simulink model "test_mdl_NI"  (R2018a)
settings: Solver=VariableStepAuto  StartTime=0.0  StopTime=10.0  RelTol=1e-3
(part 18 of 24)

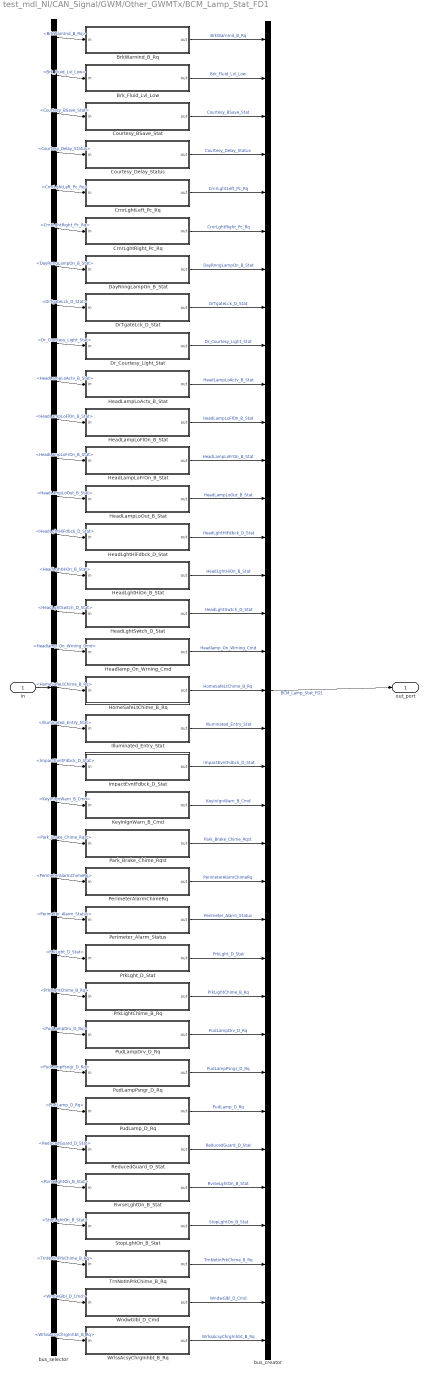
== system test_mdl_NI/CAN_Signal/GWM/Other_GWMTx/BCM_Lamp_Stat_FD1 ==
  in : Inport
  BrkWarnInd_B_Rq : Subsystem
  Brk_Fluid_Lvl_Low : Subsystem
  Courtesy_BSave_Stat : Subsystem
  Courtesy_Delay_Status : Subsystem
  CrnrLghtLeft_Pc_Rq : Subsystem
  CrnrLghtRight_Pc_Rq : Subsystem
  DayRnngLampOn_B_Stat : Subsystem
  DrTgateLck_D_Stat : Subsystem
  Dr_Courtesy_Light_Stat : Subsystem
  HeadLampLoActv_B_Stat : Subsystem
  HeadLampLoFlOn_B_Stat : Subsystem
  HeadLampLoFrOn_B_Stat : Subsystem
  HeadLampLoOut_B_Stat : Subsystem
  HeadLghtHiFdbck_D_Stat : Subsystem
  HeadLghtHiOn_B_Stat : Subsystem
  HeadLghtSwtch_D_Stat : Subsystem
  Headlamp_On_Wrning_Cmd : Subsystem
  HomeSafeLtChime_B_Rq : Subsystem
  Illuminated_Entry_Stat : Subsystem
  ImpactEvntFdbck_D_Stat : Subsystem
  KeyInIgnWarn_B_Cmd : Subsystem
  Park_Brake_Chime_Rqst : Subsystem
  PerimeterAlarmChimeRq : Subsystem
  Perimeter_Alarm_Status : Subsystem
  PrkLght_D_Stat : Subsystem
  PrkLightChime_B_Rq : Subsystem
  PudLampDrv_D_Rq : Subsystem
  PudLampPsngr_D_Rq : Subsystem
  PudLamp_D_Rq : Subsystem
  ReducedGuard_D_Stat : Subsystem
  RvrseLghtOn_B_Stat : Subsystem
  StopLghtOn_B_Stat : Subsystem
  TrnNotInPrkChime_B_Rq : Subsystem
  WndwGlbl_D_Cmd : Subsystem
  WrlssAcsyChrgInhbt_B_Rq : Subsystem
  bus_creator : BusCreator  Inputs=35
  bus_selector : BusSelector  OutputSignals=BrkWarnInd_B_Rq,Brk_Fluid_Lvl_Low,Courtesy_BSave_Stat,Courtesy_Delay_Status,CrnrLghtLeft_Pc_Rq,CrnrLghtRight_Pc_Rq,DayRnngLampOn_B_Stat,DrTgateLck_D_Stat,Dr_Courtesy_Light_Stat,HeadLampLoActv_B_Stat,HeadLampLoFlOn_B_Stat,HeadLampLoFrOn_B_Stat,HeadLampLoOut_B_Stat,HeadLghtHiFdbck_D_Stat,HeadLghtHiOn_B_Stat,HeadLghtSwtch_D_Stat,Headlamp_On_Wrning_Cmd,HomeSafeLtChime_B_Rq,Illuminated_Entry_Stat,ImpactEvntFdbck_D_Stat,KeyInIgnWarn_B_Cmd,Park_Brake_Chime_Rqst,PerimeterAlarmChimeRq,Perimeter_Alarm_Status,PrkLght_D_Stat,PrkLightChime_B_Rq,PudLampDrv_D_Rq,PudLampPsngr_D_Rq,PudLamp_D_Rq,ReducedGuard_D_Stat,RvrseLghtOn_B_Stat,StopLghtOn_B_Stat,TrnNotInPrkChime_B_Rq,WndwGlbl_D_Cmd,WrlssAcsyChrgInhbt_B_Rq
  out_port : Outport
  wires:
  bus_creator/1 -> out_port/1  "BCM_Lamp_Stat_FD1"
  BrkWarnInd_B_Rq/1(out) -> bus_creator/1  "BrkWarnInd_B_Rq"
  Brk_Fluid_Lvl_Low/1(out) -> bus_creator/2  "Brk_Fluid_Lvl_Low"
  Courtesy_BSave_Stat/1(out) -> bus_creator/3  "Courtesy_BSave_Stat"
  Courtesy_Delay_Status/1(out) -> bus_creator/4  "Courtesy_Delay_Status"
  CrnrLghtLeft_Pc_Rq/1(out) -> bus_creator/5  "CrnrLghtLeft_Pc_Rq"
  CrnrLghtRight_Pc_Rq/1(out) -> bus_creator/6  "CrnrLghtRight_Pc_Rq"
  DayRnngLampOn_B_Stat/1(out) -> bus_creator/7  "DayRnngLampOn_B_Stat"
  DrTgateLck_D_Stat/1(out) -> bus_creator/8  "DrTgateLck_D_Stat"
  Dr_Courtesy_Light_Stat/1(out) -> bus_creator/9  "Dr_Courtesy_Light_Stat"
  HeadLampLoActv_B_Stat/1(out) -> bus_creator/10  "HeadLampLoActv_B_Stat"
  HeadLampLoFlOn_B_Stat/1(out) -> bus_creator/11  "HeadLampLoFlOn_B_Stat"
  HeadLampLoFrOn_B_Stat/1(out) -> bus_creator/12  "HeadLampLoFrOn_B_Stat"
  HeadLampLoOut_B_Stat/1(out) -> bus_creator/13  "HeadLampLoOut_B_Stat"
  HeadLghtHiFdbck_D_Stat/1(out) -> bus_creator/14  "HeadLghtHiFdbck_D_Stat"
  HeadLghtHiOn_B_Stat/1(out) -> bus_creator/15  "HeadLghtHiOn_B_Stat"
  HeadLghtSwtch_D_Stat/1(out) -> bus_creator/16  "HeadLghtSwtch_D_Stat"
  Headlamp_On_Wrning_Cmd/1(out) -> bus_creator/17  "Headlamp_On_Wrning_Cmd"
  HomeSafeLtChime_B_Rq/1(out) -> bus_creator/18  "HomeSafeLtChime_B_Rq"
  Illuminated_Entry_Stat/1(out) -> bus_creator/19  "Illuminated_Entry_Stat"
  ImpactEvntFdbck_D_Stat/1(out) -> bus_creator/20  "ImpactEvntFdbck_D_Stat"
  KeyInIgnWarn_B_Cmd/1(out) -> bus_creator/21  "KeyInIgnWarn_B_Cmd"
  Park_Brake_Chime_Rqst/1(out) -> bus_creator/22  "Park_Brake_Chime_Rqst"
  PerimeterAlarmChimeRq/1(out) -> bus_creator/23  "PerimeterAlarmChimeRq"
  Perimeter_Alarm_Status/1(out) -> bus_creator/24  "Perimeter_Alarm_Status"
  PrkLght_D_Stat/1(out) -> bus_creator/25  "PrkLght_D_Stat"
  PrkLightChime_B_Rq/1(out) -> bus_creator/26  "PrkLightChime_B_Rq"
  PudLampDrv_D_Rq/1(out) -> bus_creator/27  "PudLampDrv_D_Rq"
  PudLampPsngr_D_Rq/1(out) -> bus_creator/28  "PudLampPsngr_D_Rq"
  PudLamp_D_Rq/1(out) -> bus_creator/29  "PudLamp_D_Rq"
  ReducedGuard_D_Stat/1(out) -> bus_creator/30  "ReducedGuard_D_Stat"
  RvrseLghtOn_B_Stat/1(out) -> bus_creator/31  "RvrseLghtOn_B_Stat"
  StopLghtOn_B_Stat/1(out) -> bus_creator/32  "StopLghtOn_B_Stat"
  TrnNotInPrkChime_B_Rq/1(out) -> bus_creator/33  "TrnNotInPrkChime_B_Rq"
  WndwGlbl_D_Cmd/1(out) -> bus_creator/34  "WndwGlbl_D_Cmd"
  WrlssAcsyChrgInhbt_B_Rq/1(out) -> bus_creator/35  "WrlssAcsyChrgInhbt_B_Rq"
  bus_selector/1 -> BrkWarnInd_B_Rq/1(in)  "<BrkWarnInd_B_Rq>"
  bus_selector/2 -> Brk_Fluid_Lvl_Low/1(in)  "<Brk_Fluid_Lvl_Low>"
  bus_selector/3 -> Courtesy_BSave_Stat/1(in)  "<Courtesy_BSave_Stat>"
  bus_selector/4 -> Courtesy_Delay_Status/1(in)  "<Courtesy_Delay_Status>"
  bus_selector/5 -> CrnrLghtLeft_Pc_Rq/1(in)  "<CrnrLghtLeft_Pc_Rq>"
  bus_selector/6 -> CrnrLghtRight_Pc_Rq/1(in)  "<CrnrLghtRight_Pc_Rq>"
  bus_selector/7 -> DayRnngLampOn_B_Stat/1(in)  "<DayRnngLampOn_B_Stat>"
  bus_selector/8 -> DrTgateLck_D_Stat/1(in)  "<DrTgateLck_D_Stat>"
  bus_selector/9 -> Dr_Courtesy_Light_Stat/1(in)  "<Dr_Courtesy_Light_Stat>"
  bus_selector/10 -> HeadLampLoActv_B_Stat/1(in)  "<HeadLampLoActv_B_Stat>"
  bus_selector/11 -> HeadLampLoFlOn_B_Stat/1(in)  "<HeadLampLoFlOn_B_Stat>"
  bus_selector/12 -> HeadLampLoFrOn_B_Stat/1(in)  "<HeadLampLoFrOn_B_Stat>"
  bus_selector/13 -> HeadLampLoOut_B_Stat/1(in)  "<HeadLampLoOut_B_Stat>"
  bus_selector/14 -> HeadLghtHiFdbck_D_Stat/1(in)  "<HeadLghtHiFdbck_D_Stat>"
  bus_selector/15 -> HeadLghtHiOn_B_Stat/1(in)  "<HeadLghtHiOn_B_Stat>"
  bus_selector/16 -> HeadLghtSwtch_D_Stat/1(in)  "<HeadLghtSwtch_D_Stat>"
  bus_selector/17 -> Headlamp_On_Wrning_Cmd/1(in)  "<Headlamp_On_Wrning_Cmd>"
  bus_selector/18 -> HomeSafeLtChime_B_Rq/1(in)  "<HomeSafeLtChime_B_Rq>"
  bus_selector/19 -> Illuminated_Entry_Stat/1(in)  "<Illuminated_Entry_Stat>"
  bus_selector/20 -> ImpactEvntFdbck_D_Stat/1(in)  "<ImpactEvntFdbck_D_Stat>"
  bus_selector/21 -> KeyInIgnWarn_B_Cmd/1(in)  "<KeyInIgnWarn_B_Cmd>"
  bus_selector/22 -> Park_Brake_Chime_Rqst/1(in)  "<Park_Brake_Chime_Rqst>"
  bus_selector/23 -> PerimeterAlarmChimeRq/1(in)  "<PerimeterAlarmChimeRq>"
  bus_selector/24 -> Perimeter_Alarm_Status/1(in)  "<Perimeter_Alarm_Status>"
  bus_selector/25 -> PrkLght_D_Stat/1(in)  "<PrkLght_D_Stat>"
  bus_selector/26 -> PrkLightChime_B_Rq/1(in)  "<PrkLightChime_B_Rq>"
  bus_selector/27 -> PudLampDrv_D_Rq/1(in)  "<PudLampDrv_D_Rq>"
  bus_selector/28 -> PudLampPsngr_D_Rq/1(in)  "<PudLampPsngr_D_Rq>"
  bus_selector/29 -> PudLamp_D_Rq/1(in)  "<PudLamp_D_Rq>"
  bus_selector/30 -> ReducedGuard_D_Stat/1(in)  "<ReducedGuard_D_Stat>"
  bus_selector/31 -> RvrseLghtOn_B_Stat/1(in)  "<RvrseLghtOn_B_Stat>"
  bus_selector/32 -> StopLghtOn_B_Stat/1(in)  "<StopLghtOn_B_Stat>"
  bus_selector/33 -> TrnNotInPrkChime_B_Rq/1(in)  "<TrnNotInPrkChime_B_Rq>"
  bus_selector/34 -> WndwGlbl_D_Cmd/1(in)  "<WndwGlbl_D_Cmd>"
  bus_selector/35 -> WrlssAcsyChrgInhbt_B_Rq/1(in)  "<WrlssAcsyChrgInhbt_B_Rq>"
  in/1 -> bus_selector/1

== system test_mdl_NI/CAN_Signal/GWM/Other_GWMTx/BatteryCharge_Data2_FD1 ==
  in : Inport
  ChrgCrdLck_D_Falt : Subsystem
  bus_creator : BusCreator  Inputs=1
  bus_selector : BusSelector  OutputSignals=ChrgCrdLck_D_Falt
  out_port : Outport
  wires:
  bus_creator/1 -> out_port/1  "BatteryCharge_Data2_FD1"
  ChrgCrdLck_D_Falt/1(out) -> bus_creator/1  "ChrgCrdLck_D_Falt"
  bus_selector/1 -> ChrgCrdLck_D_Falt/1(in)  "<ChrgCrdLck_D_Falt>"
  in/1 -> bus_selector/1

== system test_mdl_NI/CAN_Signal/GWM/Other_GWMTx/Battery_Mgmt_24V_FD1 ==
  in : Inport
  BattULo24Soc_Pc_Actl : Subsystem
  BattULo24State_D_Qlty : Subsystem
  BattULo24_Ah_DeltaRide : Subsystem
  BattULo24_B_Falt : Subsystem
  BattULo24_I_Actl : Subsystem
  bus_creator : BusCreator  Inputs=5
  bus_selector : BusSelector  OutputSignals=BattULo24Soc_Pc_Actl,BattULo24State_D_Qlty,BattULo24_Ah_DeltaRide,BattULo24_B_Falt,BattULo24_I_Actl
  out_port : Outport
  wires:
  bus_creator/1 -> out_port/1  "Battery_Mgmt_24V_FD1"
  BattULo24Soc_Pc_Actl/1(out) -> bus_creator/1  "BattULo24Soc_Pc_Actl"
  BattULo24State_D_Qlty/1(out) -> bus_creator/2  "BattULo24State_D_Qlty"
  BattULo24_Ah_DeltaRide/1(out) -> bus_creator/3  "BattULo24_Ah_DeltaRide"
  BattULo24_B_Falt/1(out) -> bus_creator/4  "BattULo24_B_Falt"
  BattULo24_I_Actl/1(out) -> bus_creator/5  "BattULo24_I_Actl"
  bus_selector/1 -> BattULo24Soc_Pc_Actl/1(in)  "<BattULo24Soc_Pc_Actl>"
  bus_selector/2 -> BattULo24State_D_Qlty/1(in)  "<BattULo24State_D_Qlty>"
  bus_selector/3 -> BattULo24_Ah_DeltaRide/1(in)  "<BattULo24_Ah_DeltaRide>"
  bus_selector/4 -> BattULo24_B_Falt/1(in)  "<BattULo24_B_Falt>"
  bus_selector/5 -> BattULo24_I_Actl/1(in)  "<BattULo24_I_Actl>"
  in/1 -> bus_selector/1

== system test_mdl_NI/CAN_Signal/GWM/Other_GWMTx/Battery_Mgmt_2_FD1 ==
  in : Inport
  BattULoChrg_D_Rq : Subsystem
  BattULoSrvc_T_Actl : Subsystem
  Batt_Crit_SoC_B : Subsystem
  Batt_Lo_SoC_B : Subsystem
  ChargeMode : Subsystem
  EngStrtInhbt_B_RqBatt : Subsystem
  IdleSpeedIncrease_El : Subsystem
  PeriodicElLoad_B_Stat : Subsystem
  PwSysULoFalt_D_Stat : Subsystem
  Shed_Drain_Eng_Off_B : Subsystem
  Shed_Feature_Group_ID : Subsystem
  Shed_Level_Req : Subsystem
  Shed_T_Eng_Off_B : Subsystem
  ULoRgenTestMde_B_Rq : Subsystem
  bus_creator : BusCreator  Inputs=14
  bus_selector : BusSelector  OutputSignals=BattULoChrg_D_Rq,BattULoSrvc_T_Actl,Batt_Crit_SoC_B,Batt_Lo_SoC_B,ChargeMode,EngStrtInhbt_B_RqBatt,IdleSpeedIncrease_El,PeriodicElLoad_B_Stat,PwSysULoFalt_D_Stat,Shed_Drain_Eng_Off_B,Shed_Feature_Group_ID,Shed_Level_Req,Shed_T_Eng_Off_B,ULoRgenTestMde_B_Rq
  out_port : Outport
  wires:
  bus_creator/1 -> out_port/1  "Battery_Mgmt_2_FD1"
  BattULoChrg_D_Rq/1(out) -> bus_creator/1  "BattULoChrg_D_Rq"
  BattULoSrvc_T_Actl/1(out) -> bus_creator/2  "BattULoSrvc_T_Actl"
  Batt_Crit_SoC_B/1(out) -> bus_creator/3  "Batt_Crit_SoC_B"
  Batt_Lo_SoC_B/1(out) -> bus_creator/4  "Batt_Lo_SoC_B"
  ChargeMode/1(out) -> bus_creator/5  "ChargeMode"
  EngStrtInhbt_B_RqBatt/1(out) -> bus_creator/6  "EngStrtInhbt_B_RqBatt"
  IdleSpeedIncrease_El/1(out) -> bus_creator/7  "IdleSpeedIncrease_El"
  PeriodicElLoad_B_Stat/1(out) -> bus_creator/8  "PeriodicElLoad_B_Stat"
  PwSysULoFalt_D_Stat/1(out) -> bus_creator/9  "PwSysULoFalt_D_Stat"
  Shed_Drain_Eng_Off_B/1(out) -> bus_creator/10  "Shed_Drain_Eng_Off_B"
  Shed_Feature_Group_ID/1(out) -> bus_creator/11  "Shed_Feature_Group_ID"
  Shed_Level_Req/1(out) -> bus_creator/12  "Shed_Level_Req"
  Shed_T_Eng_Off_B/1(out) -> bus_creator/13  "Shed_T_Eng_Off_B"
  ULoRgenTestMde_B_Rq/1(out) -> bus_creator/14  "ULoRgenTestMde_B_Rq"
  bus_selector/1 -> BattULoChrg_D_Rq/1(in)  "<BattULoChrg_D_Rq>"
  bus_selector/2 -> BattULoSrvc_T_Actl/1(in)  "<BattULoSrvc_T_Actl>"
  bus_selector/3 -> Batt_Crit_SoC_B/1(in)  "<Batt_Crit_SoC_B>"
  bus_selector/4 -> Batt_Lo_SoC_B/1(in)  "<Batt_Lo_SoC_B>"
  bus_selector/5 -> ChargeMode/1(in)  "<ChargeMode>"
  bus_selector/6 -> EngStrtInhbt_B_RqBatt/1(in)  "<EngStrtInhbt_B_RqBatt>"
  bus_selector/7 -> IdleSpeedIncrease_El/1(in)  "<IdleSpeedIncrease_El>"
  bus_selector/8 -> PeriodicElLoad_B_Stat/1(in)  "<PeriodicElLoad_B_Stat>"
  bus_selector/9 -> PwSysULoFalt_D_Stat/1(in)  "<PwSysULoFalt_D_Stat>"
  bus_selector/10 -> Shed_Drain_Eng_Off_B/1(in)  "<Shed_Drain_Eng_Off_B>"
  bus_selector/11 -> Shed_Feature_Group_ID/1(in)  "<Shed_Feature_Group_ID>"
  bus_selector/12 -> Shed_Level_Req/1(in)  "<Shed_Level_Req>"
  bus_selector/13 -> Shed_T_Eng_Off_B/1(in)  "<Shed_T_Eng_Off_B>"
  bus_selector/14 -> ULoRgenTestMde_B_Rq/1(in)  "<ULoRgenTestMde_B_Rq>"
  in/1 -> bus_selector/1

== system test_mdl_NI/CAN_Signal/GWM/Other_GWMTx/Battery_Mgmt_3_FD1 ==
  in : Inport
  BSBattQCapAh : Subsystem
  BSBattQDeltaRideAh : Subsystem
  BSBattSOC : Subsystem
  BSFault : Subsystem
  BattULo2_Te_Actl : Subsystem
  BattULoChrg_URate_RqMx : Subsystem
  BattULoChrg_U_RqMn : Subsystem
  BattULoChrg_U_RqMx : Subsystem
  BattULoState_D_Qlty : Subsystem
  bus_creator : BusCreator  Inputs=9
  bus_selector : BusSelector  OutputSignals=BSBattQCapAh,BSBattQDeltaRideAh,BSBattSOC,BSFault,BattULo2_Te_Actl,BattULoChrg_URate_RqMx,BattULoChrg_U_RqMn,BattULoChrg_U_RqMx,BattULoState_D_Qlty
  out_port : Outport
  wires:
  bus_creator/1 -> out_port/1  "Battery_Mgmt_3_FD1"
  BSBattQCapAh/1(out) -> bus_creator/1  "BSBattQCapAh"
  BSBattQDeltaRideAh/1(out) -> bus_creator/2  "BSBattQDeltaRideAh"
  BSBattSOC/1(out) -> bus_creator/3  "BSBattSOC"
  BSFault/1(out) -> bus_creator/4  "BSFault"
  BattULo2_Te_Actl/1(out) -> bus_creator/5  "BattULo2_Te_Actl"
  BattULoChrg_URate_RqMx/1(out) -> bus_creator/6  "BattULoChrg_URate_RqMx"
  BattULoChrg_U_RqMn/1(out) -> bus_creator/7  "BattULoChrg_U_RqMn"
  BattULoChrg_U_RqMx/1(out) -> bus_creator/8  "BattULoChrg_U_RqMx"
  BattULoState_D_Qlty/1(out) -> bus_creator/9  "BattULoState_D_Qlty"
  bus_selector/1 -> BSBattQCapAh/1(in)  "<BSBattQCapAh>"
  bus_selector/2 -> BSBattQDeltaRideAh/1(in)  "<BSBattQDeltaRideAh>"
  bus_selector/3 -> BSBattSOC/1(in)  "<BSBattSOC>"
  bus_selector/4 -> BSFault/1(in)  "<BSFault>"
  bus_selector/5 -> BattULo2_Te_Actl/1(in)  "<BattULo2_Te_Actl>"
  bus_selector/6 -> BattULoChrg_URate_RqMx/1(in)  "<BattULoChrg_URate_RqMx>"
  bus_selector/7 -> BattULoChrg_U_RqMn/1(in)  "<BattULoChrg_U_RqMn>"
  bus_selector/8 -> BattULoChrg_U_RqMx/1(in)  "<BattULoChrg_U_RqMx>"
  bus_selector/9 -> BattULoState_D_Qlty/1(in)  "<BattULoState_D_Qlty>"
  in/1 -> bus_selector/1

== system test_mdl_NI/CAN_Signal/GWM/Other_GWMTx/Battery_Mgmt_4_FD1 ==
  in : Inport
  BattULoAuxSoc_Pc_Actl : Subsystem
  BattULoAux_B_Falt : Subsystem
  BattULoAux_D_Qlty : Subsystem
  BattULoAux_I_Actl : Subsystem
  BattULoAux_U_Actl : Subsystem
  BattULoCrnkBelt_U_Pred : Subsystem
  BattULoCrnkStrt_U_Pred : Subsystem
  bus_creator : BusCreator  Inputs=7
  bus_selector : BusSelector  OutputSignals=BattULoAuxSoc_Pc_Actl,BattULoAux_B_Falt,BattULoAux_D_Qlty,BattULoAux_I_Actl,BattULoAux_U_Actl,BattULoCrnkBelt_U_Pred,BattULoCrnkStrt_U_Pred
  out_port : Outport
  wires:
  bus_creator/1 -> out_port/1  "Battery_Mgmt_4_FD1"
  BattULoAuxSoc_Pc_Actl/1(out) -> bus_creator/1  "BattULoAuxSoc_Pc_Actl"
  BattULoAux_B_Falt/1(out) -> bus_creator/2  "BattULoAux_B_Falt"
  BattULoAux_D_Qlty/1(out) -> bus_creator/3  "BattULoAux_D_Qlty"
  BattULoAux_I_Actl/1(out) -> bus_creator/4  "BattULoAux_I_Actl"
  BattULoAux_U_Actl/1(out) -> bus_creator/5  "BattULoAux_U_Actl"
  BattULoCrnkBelt_U_Pred/1(out) -> bus_creator/6  "BattULoCrnkBelt_U_Pred"
  BattULoCrnkStrt_U_Pred/1(out) -> bus_creator/7  "BattULoCrnkStrt_U_Pred"
  bus_selector/1 -> BattULoAuxSoc_Pc_Actl/1(in)  "<BattULoAuxSoc_Pc_Actl>"
  bus_selector/2 -> BattULoAux_B_Falt/1(in)  "<BattULoAux_B_Falt>"
  bus_selector/3 -> BattULoAux_D_Qlty/1(in)  "<BattULoAux_D_Qlty>"
  bus_selector/4 -> BattULoAux_I_Actl/1(in)  "<BattULoAux_I_Actl>"
  bus_selector/5 -> BattULoAux_U_Actl/1(in)  "<BattULoAux_U_Actl>"
  bus_selector/6 -> BattULoCrnkBelt_U_Pred/1(in)  "<BattULoCrnkBelt_U_Pred>"
  bus_selector/7 -> BattULoCrnkStrt_U_Pred/1(in)  "<BattULoCrnkStrt_U_Pred>"
  in/1 -> bus_selector/1

== system test_mdl_NI/CAN_Signal/GWM/Other_GWMTx/Battery_Traction_1_FD1 ==
  in : Inport
  BattTracMil_D_Rq : Subsystem
  BattTracOffFst_D_Actl : Subsystem
  BattTracOff_B_Actl : Subsystem
  BattTrac_I_Actl : Subsystem
  BattTrac_U_Actl : Subsystem
  BattTrac_U_LimHi : Subsystem
  BattTrac_U_LimLo : Subsystem
  VehStrtInhbt_B_RqBatt : Subsystem
  bus_creator : BusCreator  Inputs=8
  bus_selector : BusSelector  OutputSignals=BattTracMil_D_Rq,BattTracOffFst_D_Actl,BattTracOff_B_Actl,BattTrac_I_Actl,BattTrac_U_Actl,BattTrac_U_LimHi,BattTrac_U_LimLo,VehStrtInhbt_B_RqBatt
  out_port : Outport
  wires:
  bus_creator/1 -> out_port/1  "Battery_Traction_1_FD1"
  BattTracMil_D_Rq/1(out) -> bus_creator/1  "BattTracMil_D_Rq"
  BattTracOffFst_D_Actl/1(out) -> bus_creator/2  "BattTracOffFst_D_Actl"
  BattTracOff_B_Actl/1(out) -> bus_creator/3  "BattTracOff_B_Actl"
  BattTrac_I_Actl/1(out) -> bus_creator/4  "BattTrac_I_Actl"
  BattTrac_U_Actl/1(out) -> bus_creator/5  "BattTrac_U_Actl"
  BattTrac_U_LimHi/1(out) -> bus_creator/6  "BattTrac_U_LimHi"
  BattTrac_U_LimLo/1(out) -> bus_creator/7  "BattTrac_U_LimLo"
  VehStrtInhbt_B_RqBatt/1(out) -> bus_creator/8  "VehStrtInhbt_B_RqBatt"
  bus_selector/1 -> BattTracMil_D_Rq/1(in)  "<BattTracMil_D_Rq>"
  bus_selector/2 -> BattTracOffFst_D_Actl/1(in)  "<BattTracOffFst_D_Actl>"
  bus_selector/3 -> BattTracOff_B_Actl/1(in)  "<BattTracOff_B_Actl>"
  bus_selector/4 -> BattTrac_I_Actl/1(in)  "<BattTrac_I_Actl>"
  bus_selector/5 -> BattTrac_U_Actl/1(in)  "<BattTrac_U_Actl>"
  bus_selector/6 -> BattTrac_U_LimHi/1(in)  "<BattTrac_U_LimHi>"
  bus_selector/7 -> BattTrac_U_LimLo/1(in)  "<BattTrac_U_LimLo>"
  bus_selector/8 -> VehStrtInhbt_B_RqBatt/1(in)  "<VehStrtInhbt_B_RqBatt>"
  in/1 -> bus_selector/1

== system test_mdl_NI/CAN_Signal/GWM/Other_GWMTx/Battery_Traction_3_FD1 ==
  in : Inport
  BattTracClnt_Te_Actl : Subsystem
  BattTracSoc_Pc_LimHi : Subsystem
  BattTracSoc_Pc_LimLo : Subsystem
  BattTracSoc_Pc_MnPrtct : Subsystem
  BattTracSoc_Pc_MxPrtct : Subsystem
  BattTracSrvcRqd_B_Rq : Subsystem
  BattTracWarnLamp_B_Rq : Subsystem
  bus_creator : BusCreator  Inputs=7
  bus_selector : BusSelector  OutputSignals=BattTracClnt_Te_Actl,BattTracSoc_Pc_LimHi,BattTracSoc_Pc_LimLo,BattTracSoc_Pc_MnPrtct,BattTracSoc_Pc_MxPrtct,BattTracSrvcRqd_B_Rq,BattTracWarnLamp_B_Rq
  out_port : Outport
  wires:
  bus_creator/1 -> out_port/1  "Battery_Traction_3_FD1"
  BattTracClnt_Te_Actl/1(out) -> bus_creator/1  "BattTracClnt_Te_Actl"
  BattTracSoc_Pc_LimHi/1(out) -> bus_creator/2  "BattTracSoc_Pc_LimHi"
  BattTracSoc_Pc_LimLo/1(out) -> bus_creator/3  "BattTracSoc_Pc_LimLo"
  BattTracSoc_Pc_MnPrtct/1(out) -> bus_creator/4  "BattTracSoc_Pc_MnPrtct"
  BattTracSoc_Pc_MxPrtct/1(out) -> bus_creator/5  "BattTracSoc_Pc_MxPrtct"
  BattTracSrvcRqd_B_Rq/1(out) -> bus_creator/6  "BattTracSrvcRqd_B_Rq"
  BattTracWarnLamp_B_Rq/1(out) -> bus_creator/7  "BattTracWarnLamp_B_Rq"
  bus_selector/1 -> BattTracClnt_Te_Actl/1(in)  "<BattTracClnt_Te_Actl>"
  bus_selector/2 -> BattTracSoc_Pc_LimHi/1(in)  "<BattTracSoc_Pc_LimHi>"
  bus_selector/3 -> BattTracSoc_Pc_LimLo/1(in)  "<BattTracSoc_Pc_LimLo>"
  bus_selector/4 -> BattTracSoc_Pc_MnPrtct/1(in)  "<BattTracSoc_Pc_MnPrtct>"
  bus_selector/5 -> BattTracSoc_Pc_MxPrtct/1(in)  "<BattTracSoc_Pc_MxPrtct>"
  bus_selector/6 -> BattTracSrvcRqd_B_Rq/1(in)  "<BattTracSrvcRqd_B_Rq>"
  bus_selector/7 -> BattTracWarnLamp_B_Rq/1(in)  "<BattTracWarnLamp_B_Rq>"
  in/1 -> bus_selector/1

== system test_mdl_NI/CAN_Signal/GWM/Other_GWMTx/Battery_Traction_4_FD1 ==
  in : Inport
  BattTracDiagClr_B_Rq : Subsystem
  BattTracSoc2_Pc_Actl : Subsystem
  BattTrac_Te_Actl : Subsystem
  bus_creator : BusCreator  Inputs=3
  bus_selector : BusSelector  OutputSignals=BattTracDiagClr_B_Rq,BattTracSoc2_Pc_Actl,BattTrac_Te_Actl
  out_port : Outport
  wires:
  bus_creator/1 -> out_port/1  "Battery_Traction_4_FD1"
  BattTracDiagClr_B_Rq/1(out) -> bus_creator/1  "BattTracDiagClr_B_Rq"
  BattTracSoc2_Pc_Actl/1(out) -> bus_creator/2  "BattTracSoc2_Pc_Actl"
  BattTrac_Te_Actl/1(out) -> bus_creator/3  "BattTrac_Te_Actl"
  bus_selector/1 -> BattTracDiagClr_B_Rq/1(in)  "<BattTracDiagClr_B_Rq>"
  bus_selector/2 -> BattTracSoc2_Pc_Actl/1(in)  "<BattTracSoc2_Pc_Actl>"
  bus_selector/3 -> BattTrac_Te_Actl/1(in)  "<BattTrac_Te_Actl>"
  in/1 -> bus_selector/1

== system test_mdl_NI/CAN_Signal/GWM/Other_GWMTx/Battery_Traction_5_FD1 ==
  in : Inport
  BattTrac2_Pw_ChrgInst : Subsystem
  BattTrac2_Pw_DchrgInst : Subsystem
  BattTrac2_Pw_LimChrg : Subsystem
  BattTrac2_Pw_LimDchrg : Subsystem
  bus_creator : BusCreator  Inputs=4
  bus_selector : BusSelector  OutputSignals=BattTrac2_Pw_ChrgInst,BattTrac2_Pw_DchrgInst,BattTrac2_Pw_LimChrg,BattTrac2_Pw_LimDchrg
  out_port : Outport
  wires:
  bus_creator/1 -> out_port/1  "Battery_Traction_5_FD1"
  BattTrac2_Pw_ChrgInst/1(out) -> bus_creator/1  "BattTrac2_Pw_ChrgInst"
  BattTrac2_Pw_DchrgInst/1(out) -> bus_creator/2  "BattTrac2_Pw_DchrgInst"
  BattTrac2_Pw_LimChrg/1(out) -> bus_creator/3  "BattTrac2_Pw_LimChrg"
  BattTrac2_Pw_LimDchrg/1(out) -> bus_creator/4  "BattTrac2_Pw_LimDchrg"
  bus_selector/1 -> BattTrac2_Pw_ChrgInst/1(in)  "<BattTrac2_Pw_ChrgInst>"
  bus_selector/2 -> BattTrac2_Pw_DchrgInst/1(in)  "<BattTrac2_Pw_DchrgInst>"
  bus_selector/3 -> BattTrac2_Pw_LimChrg/1(in)  "<BattTrac2_Pw_LimChrg>"
  bus_selector/4 -> BattTrac2_Pw_LimDchrg/1(in)  "<BattTrac2_Pw_LimDchrg>"
  in/1 -> bus_selector/1

== system test_mdl_NI/CAN_Signal/GWM/Other_GWMTx/Battery_Traction_6_FD1 ==
  in : Inport
  BattTracClntPmp_D_Stat : Subsystem
  BattTracCnnct_D_Cmd : Subsystem
  BattTracDcdcDis_B_Rq : Subsystem
  BattTracDelta_Te_Actl : Subsystem
  BattTracHvilOpen_B_Stat : Subsystem
  HtrnClntPump_D_Stat : Subsystem
  bus_creator : BusCreator  Inputs=6
  bus_selector : BusSelector  OutputSignals=BattTracClntPmp_D_Stat,BattTracCnnct_D_Cmd,BattTracDcdcDis_B_Rq,BattTracDelta_Te_Actl,BattTracHvilOpen_B_Stat,HtrnClntPump_D_Stat
  out_port : Outport
  wires:
  bus_creator/1 -> out_port/1  "Battery_Traction_6_FD1"
  BattTracClntPmp_D_Stat/1(out) -> bus_creator/1  "BattTracClntPmp_D_Stat"
  BattTracCnnct_D_Cmd/1(out) -> bus_creator/2  "BattTracCnnct_D_Cmd"
  BattTracDcdcDis_B_Rq/1(out) -> bus_creator/3  "BattTracDcdcDis_B_Rq"
  BattTracDelta_Te_Actl/1(out) -> bus_creator/4  "BattTracDelta_Te_Actl"
  BattTracHvilOpen_B_Stat/1(out) -> bus_creator/5  "BattTracHvilOpen_B_Stat"
  HtrnClntPump_D_Stat/1(out) -> bus_creator/6  "HtrnClntPump_D_Stat"
  bus_selector/1 -> BattTracClntPmp_D_Stat/1(in)  "<BattTracClntPmp_D_Stat>"
  bus_selector/2 -> BattTracCnnct_D_Cmd/1(in)  "<BattTracCnnct_D_Cmd>"
  bus_selector/3 -> BattTracDcdcDis_B_Rq/1(in)  "<BattTracDcdcDis_B_Rq>"
  bus_selector/4 -> BattTracDelta_Te_Actl/1(in)  "<BattTracDelta_Te_Actl>"
  bus_selector/5 -> BattTracHvilOpen_B_Stat/1(in)  "<BattTracHvilOpen_B_Stat>"
  bus_selector/6 -> HtrnClntPump_D_Stat/1(in)  "<HtrnClntPump_D_Stat>"
  in/1 -> bus_selector/1

== system test_mdl_NI/CAN_Signal/GWM/Other_GWMTx/BodyInfo_3_FD1 ==
  in : Inport
  Backlit_LED_Status : Subsystem
  BodySrvcRqd_B_Rq : Subsystem
  CrashEvnt_D_Stat : Subsystem
  Day_Night_Status : Subsystem
  Delay_Accy : Subsystem
  DimmingLvlEvnt_No_Actl : Subsystem
  Dimming_Lvl : Subsystem
  DrStatDrvErrCnt_B_Stat : Subsystem
  DrStatDrv_B_Actl : Subsystem
  DrStatHood_B_Actl : Subsystem
  DrStatInnrTgate_B_Actl : Subsystem
  DrStatPsngr_B_Actl : Subsystem
  DrStatRl_B_Actl : Subsystem
  DrStatRr_B_Actl : Subsystem
  DrStatTgate_B_Actl : Subsystem
  FogLghtFrontOn_B_Stat : Subsystem
  FogLghtRearOn_B_Stat : Subsystem
  FuelPmpInhbt_B_Stat : Subsystem
  IgnKeyType_D_Actl : Subsystem
  Ignition_Status : Subsystem
  Key_In_Ignition_Stat : Subsystem
  LifeCycMde_D_Actl : Subsystem
  Litval : Subsystem
  Parklamp_Status : Subsystem
  PrkBrkActv_B_Actl : Subsystem
  Remote_Start_Status : Subsystem
  TurnLghtLeftOn_B_Stat : Subsystem
  TurnLghtLeft_D_Rq : Subsystem
  TurnLghtRightOn_B_Stat : Subsystem
  TurnLghtRight_D_Rq : Subsystem
  ValetMode_D_Mem : Subsystem
  bus_creator : BusCreator  Inputs=31
  bus_selector : BusSelector  OutputSignals=Backlit_LED_Status,BodySrvcRqd_B_Rq,CrashEvnt_D_Stat,Day_Night_Status,Delay_Accy,DimmingLvlEvnt_No_Actl,Dimming_Lvl,DrStatDrvErrCnt_B_Stat,DrStatDrv_B_Actl,DrStatHood_B_Actl,DrStatInnrTgate_B_Actl,DrStatPsngr_B_Actl,DrStatRl_B_Actl,DrStatRr_B_Actl,DrStatTgate_B_Actl,FogLghtFrontOn_B_Stat,FogLghtRearOn_B_Stat,FuelPmpInhbt_B_Stat,IgnKeyType_D_Actl,Ignition_Status,Key_In_Ignition_Stat,LifeCycMde_D_Actl,Litval,Parklamp_Status,PrkBrkActv_B_Actl,Remote_Start_Status,TurnLghtLeftOn_B_Stat,TurnLghtLeft_D_Rq,TurnLghtRightOn_B_Stat,TurnLghtRight_D_Rq,ValetMode_D_Mem
  out_port : Outport
  wires:
  bus_creator/1 -> out_port/1  "BodyInfo_3_FD1"
  Backlit_LED_Status/1(out) -> bus_creator/1  "Backlit_LED_Status"
  BodySrvcRqd_B_Rq/1(out) -> bus_creator/2  "BodySrvcRqd_B_Rq"
  CrashEvnt_D_Stat/1(out) -> bus_creator/3  "CrashEvnt_D_Stat"
  Day_Night_Status/1(out) -> bus_creator/4  "Day_Night_Status"
  Delay_Accy/1(out) -> bus_creator/5  "Delay_Accy"
  DimmingLvlEvnt_No_Actl/1(out) -> bus_creator/6  "DimmingLvlEvnt_No_Actl"
  Dimming_Lvl/1(out) -> bus_creator/7  "Dimming_Lvl"
  DrStatDrvErrCnt_B_Stat/1(out) -> bus_creator/8  "DrStatDrvErrCnt_B_Stat"
  DrStatDrv_B_Actl/1(out) -> bus_creator/9  "DrStatDrv_B_Actl"
  DrStatHood_B_Actl/1(out) -> bus_creator/10  "DrStatHood_B_Actl"
  DrStatInnrTgate_B_Actl/1(out) -> bus_creator/11  "DrStatInnrTgate_B_Actl"
  DrStatPsngr_B_Actl/1(out) -> bus_creator/12  "DrStatPsngr_B_Actl"
  DrStatRl_B_Actl/1(out) -> bus_creator/13  "DrStatRl_B_Actl"
  DrStatRr_B_Actl/1(out) -> bus_creator/14  "DrStatRr_B_Actl"
  DrStatTgate_B_Actl/1(out) -> bus_creator/15  "DrStatTgate_B_Actl"
  FogLghtFrontOn_B_Stat/1(out) -> bus_creator/16  "FogLghtFrontOn_B_Stat"
  FogLghtRearOn_B_Stat/1(out) -> bus_creator/17  "FogLghtRearOn_B_Stat"
  FuelPmpInhbt_B_Stat/1(out) -> bus_creator/18  "FuelPmpInhbt_B_Stat"
  IgnKeyType_D_Actl/1(out) -> bus_creator/19  "IgnKeyType_D_Actl"
  Ignition_Status/1(out) -> bus_creator/20  "Ignition_Status"
  Key_In_Ignition_Stat/1(out) -> bus_creator/21  "Key_In_Ignition_Stat"
  LifeCycMde_D_Actl/1(out) -> bus_creator/22  "LifeCycMde_D_Actl"
  Litval/1(out) -> bus_creator/23  "Litval"
  Parklamp_Status/1(out) -> bus_creator/24  "Parklamp_Status"
  PrkBrkActv_B_Actl/1(out) -> bus_creator/25  "PrkBrkActv_B_Actl"
  Remote_Start_Status/1(out) -> bus_creator/26  "Remote_Start_Status"
  TurnLghtLeftOn_B_Stat/1(out) -> bus_creator/27  "TurnLghtLeftOn_B_Stat"
  TurnLghtLeft_D_Rq/1(out) -> bus_creator/28  "TurnLghtLeft_D_Rq"
  TurnLghtRightOn_B_Stat/1(out) -> bus_creator/29  "TurnLghtRightOn_B_Stat"
  TurnLghtRight_D_Rq/1(out) -> bus_creator/30  "TurnLghtRight_D_Rq"
  ValetMode_D_Mem/1(out) -> bus_creator/31  "ValetMode_D_Mem"
  bus_selector/1 -> Backlit_LED_Status/1(in)  "<Backlit_LED_Status>"
  bus_selector/2 -> BodySrvcRqd_B_Rq/1(in)  "<BodySrvcRqd_B_Rq>"
  bus_selector/3 -> CrashEvnt_D_Stat/1(in)  "<CrashEvnt_D_Stat>"
  bus_selector/4 -> Day_Night_Status/1(in)  "<Day_Night_Status>"
  bus_selector/5 -> Delay_Accy/1(in)  "<Delay_Accy>"
  bus_selector/6 -> DimmingLvlEvnt_No_Actl/1(in)  "<DimmingLvlEvnt_No_Actl>"
  bus_selector/7 -> Dimming_Lvl/1(in)  "<Dimming_Lvl>"
  bus_selector/8 -> DrStatDrvErrCnt_B_Stat/1(in)  "<DrStatDrvErrCnt_B_Stat>"
  bus_selector/9 -> DrStatDrv_B_Actl/1(in)  "<DrStatDrv_B_Actl>"
  bus_selector/10 -> DrStatHood_B_Actl/1(in)  "<DrStatHood_B_Actl>"
  bus_selector/11 -> DrStatInnrTgate_B_Actl/1(in)  "<DrStatInnrTgate_B_Actl>"
  bus_selector/12 -> DrStatPsngr_B_Actl/1(in)  "<DrStatPsngr_B_Actl>"
  bus_selector/13 -> DrStatRl_B_Actl/1(in)  "<DrStatRl_B_Actl>"
  bus_selector/14 -> DrStatRr_B_Actl/1(in)  "<DrStatRr_B_Actl>"
  bus_selector/15 -> DrStatTgate_B_Actl/1(in)  "<DrStatTgate_B_Actl>"
  bus_selector/16 -> FogLghtFrontOn_B_Stat/1(in)  "<FogLghtFrontOn_B_Stat>"
  bus_selector/17 -> FogLghtRearOn_B_Stat/1(in)  "<FogLghtRearOn_B_Stat>"
  bus_selector/18 -> FuelPmpInhbt_B_Stat/1(in)  "<FuelPmpInhbt_B_Stat>"
  bus_selector/19 -> IgnKeyType_D_Actl/1(in)  "<IgnKeyType_D_Actl>"
  bus_selector/20 -> Ignition_Status/1(in)  "<Ignition_Status>"
  bus_selector/21 -> Key_In_Ignition_Stat/1(in)  "<Key_In_Ignition_Stat>"
  bus_selector/22 -> LifeCycMde_D_Actl/1(in)  "<LifeCycMde_D_Actl>"
  bus_selector/23 -> Litval/1(in)  "<Litval>"
  bus_selector/24 -> Parklamp_Status/1(in)  "<Parklamp_Status>"
  bus_selector/25 -> PrkBrkActv_B_Actl/1(in)  "<PrkBrkActv_B_Actl>"
  bus_selector/26 -> Remote_Start_Status/1(in)  "<Remote_Start_Status>"
  bus_selector/27 -> TurnLghtLeftOn_B_Stat/1(in)  "<TurnLghtLeftOn_B_Stat>"
  bus_selector/28 -> TurnLghtLeft_D_Rq/1(in)  "<TurnLghtLeft_D_Rq>"
  bus_selector/29 -> TurnLghtRightOn_B_Stat/1(in)  "<TurnLghtRightOn_B_Stat>"
  bus_selector/30 -> TurnLghtRight_D_Rq/1(in)  "<TurnLghtRight_D_Rq>"
  bus_selector/31 -> ValetMode_D_Mem/1(in)  "<ValetMode_D_Mem>"
  in/1 -> bus_selector/1

== system test_mdl_NI/CAN_Signal/GWM/Other_GWMTx/Body_Info_10_FD1 ==
  in : Inport
  GenericSwtch1_No_Actl : Subsystem
  GenericSwtch2_No_Actl : Subsystem
  GenericSwtch3_No_Actl : Subsystem
  bus_creator : BusCreator  Inputs=3
  bus_selector : BusSelector  OutputSignals=GenericSwtch1_No_Actl,GenericSwtch2_No_Actl,GenericSwtch3_No_Actl
  out_port : Outport
  wires:
  bus_creator/1 -> out_port/1  "Body_Info_10_FD1"
  GenericSwtch1_No_Actl/1(out) -> bus_creator/1  "GenericSwtch1_No_Actl"
  GenericSwtch2_No_Actl/1(out) -> bus_creator/2  "GenericSwtch2_No_Actl"
  GenericSwtch3_No_Actl/1(out) -> bus_creator/3  "GenericSwtch3_No_Actl"
  bus_selector/1 -> GenericSwtch1_No_Actl/1(in)  "<GenericSwtch1_No_Actl>"
  bus_selector/2 -> GenericSwtch2_No_Actl/1(in)  "<GenericSwtch2_No_Actl>"
  bus_selector/3 -> GenericSwtch3_No_Actl/1(in)  "<GenericSwtch3_No_Actl>"
  in/1 -> bus_selector/1

== system test_mdl_NI/CAN_Signal/GWM/Other_GWMTx/Body_Info_4_FD1 ==
  in : Inport
  BattULo_I_Actl : Subsystem
  BattULo_U_Actl : Subsystem
  BrkTrnShifLck_B_Stat : Subsystem
  DcacElPw_D_Rq : Subsystem
  DriverCrankingReq : Subsystem
  EngOff_T_Actl : Subsystem
  FuelPumpPwr_D_Stat : Subsystem
  PrkLckCtlAvail_T_Stat : Subsystem
  PrkLckCtlMsgTxt_D_Rq : Subsystem
  PrkLckCtlTow_B_Enbl : Subsystem
  PrkLckCtlUnlck_D_Stat : Subsystem
  PrkLckCtl_B_Enbl : Subsystem
  PtLatchActv_B_RqBcm : Subsystem
  ReFuelSwtchStat_D_Actl : Subsystem
  bus_creator : BusCreator  Inputs=15
  bus_selector : BusSelector  OutputSignals=BattULo_I_Actl,BattULo_U_Actl,BrkTrnShifLck_B_Stat,DcacElPw_D_Rq,DriverCrankingReq,EngOff_T_Actl,FuelPumpPwr_D_Stat,PrkLckCtlAvail_T_Stat,PrkLckCtlMsgTxt_D_Rq,PrkLckCtlTow_B_Enbl,PrkLckCtlUnlck_D_Stat,PrkLckCtl_B_Enbl,PtLatchActv_B_RqBcm,ReFuelSwtchStat_D_Actl,immoSecureIdleMode
  immoSecureIdleMode : Subsystem
  out_port : Outport
  wires:
  bus_creator/1 -> out_port/1  "Body_Info_4_FD1"
  BattULo_I_Actl/1(out) -> bus_creator/1  "BattULo_I_Actl"
  BattULo_U_Actl/1(out) -> bus_creator/2  "BattULo_U_Actl"
  BrkTrnShifLck_B_Stat/1(out) -> bus_creator/3  "BrkTrnShifLck_B_Stat"
  DcacElPw_D_Rq/1(out) -> bus_creator/4  "DcacElPw_D_Rq"
  DriverCrankingReq/1(out) -> bus_creator/5  "DriverCrankingReq"
  EngOff_T_Actl/1(out) -> bus_creator/6  "EngOff_T_Actl"
  FuelPumpPwr_D_Stat/1(out) -> bus_creator/7  "FuelPumpPwr_D_Stat"
  PrkLckCtlAvail_T_Stat/1(out) -> bus_creator/8  "PrkLckCtlAvail_T_Stat"
  PrkLckCtlMsgTxt_D_Rq/1(out) -> bus_creator/9  "PrkLckCtlMsgTxt_D_Rq"
  PrkLckCtlTow_B_Enbl/1(out) -> bus_creator/10  "PrkLckCtlTow_B_Enbl"
  PrkLckCtlUnlck_D_Stat/1(out) -> bus_creator/11  "PrkLckCtlUnlck_D_Stat"
  PrkLckCtl_B_Enbl/1(out) -> bus_creator/12  "PrkLckCtl_B_Enbl"
  PtLatchActv_B_RqBcm/1(out) -> bus_creator/13  "PtLatchActv_B_RqBcm"
  ReFuelSwtchStat_D_Actl/1(out) -> bus_creator/14  "ReFuelSwtchStat_D_Actl"
  immoSecureIdleMode/1(out) -> bus_creator/15  "immoSecureIdleMode"
  bus_selector/1 -> BattULo_I_Actl/1(in)  "<BattULo_I_Actl>"
  bus_selector/2 -> BattULo_U_Actl/1(in)  "<BattULo_U_Actl>"
  bus_selector/3 -> BrkTrnShifLck_B_Stat/1(in)  "<BrkTrnShifLck_B_Stat>"
  bus_selector/4 -> DcacElPw_D_Rq/1(in)  "<DcacElPw_D_Rq>"
  bus_selector/5 -> DriverCrankingReq/1(in)  "<DriverCrankingReq>"
  bus_selector/6 -> EngOff_T_Actl/1(in)  "<EngOff_T_Actl>"
  bus_selector/7 -> FuelPumpPwr_D_Stat/1(in)  "<FuelPumpPwr_D_Stat>"
  bus_selector/8 -> PrkLckCtlAvail_T_Stat/1(in)  "<PrkLckCtlAvail_T_Stat>"
  bus_selector/9 -> PrkLckCtlMsgTxt_D_Rq/1(in)  "<PrkLckCtlMsgTxt_D_Rq>"
  bus_selector/10 -> PrkLckCtlTow_B_Enbl/1(in)  "<PrkLckCtlTow_B_Enbl>"
  bus_selector/11 -> PrkLckCtlUnlck_D_Stat/1(in)  "<PrkLckCtlUnlck_D_Stat>"
  bus_selector/12 -> PrkLckCtl_B_Enbl/1(in)  "<PrkLckCtl_B_Enbl>"
  bus_selector/13 -> PtLatchActv_B_RqBcm/1(in)  "<PtLatchActv_B_RqBcm>"
  bus_selector/14 -> ReFuelSwtchStat_D_Actl/1(in)  "<ReFuelSwtchStat_D_Actl>"
  bus_selector/15 -> immoSecureIdleMode/1(in)  "<immoSecureIdleMode>"
  in/1 -> bus_selector/1

== system test_mdl_NI/CAN_Signal/GWM/Other_GWMTx/Body_Info_6_FD1 ==
  in : Inport
  DrLatchMsgTxt_D_Rq : Subsystem
  ElPwPoint_D_Rq : Subsystem
  HeadLghtHiPrmsn_D_Stat : Subsystem
  IgnPsswrdDsply_B_Rq : Subsystem
  KeyAdmnTot_No_Cnt : Subsystem
  KeyMykeyTot_No_Cnt : Subsystem
  Keycode_Status : Subsystem
  PEBackupSlot_Stats : Subsystem
  PoliceIdlMde_D_Stat : Subsystem
  PrmtrAlrmEvnt_D_Stat : Subsystem
  PrsnlDevcChrgEnbl_B_Rq : Subsystem
  SecurityMsgTxt_D_Rq : Subsystem
  SteWhlLckMsgTxt_D_Rq : Subsystem
  TracKeyMde_D_Stat : Subsystem
  bus_creator : BusCreator  Inputs=15
  bus_selector : BusSelector  OutputSignals=DrLatchMsgTxt_D_Rq,ElPwPoint_D_Rq,HeadLghtHiPrmsn_D_Stat,IgnPsswrdDsply_B_Rq,KeyAdmnTot_No_Cnt,KeyMykeyTot_No_Cnt,Keycode_Status,PEBackupSlot_Stats,PoliceIdlMde_D_Stat,PrmtrAlrmEvnt_D_Stat,PrsnlDevcChrgEnbl_B_Rq,SecurityMsgTxt_D_Rq,SteWhlLckMsgTxt_D_Rq,TracKeyMde_D_Stat,immoMsgTxt_D_Rq
  immoMsgTxt_D_Rq : Subsystem
  out_port : Outport
  wires:
  bus_creator/1 -> out_port/1  "Body_Info_6_FD1"
  DrLatchMsgTxt_D_Rq/1(out) -> bus_creator/1  "DrLatchMsgTxt_D_Rq"
  ElPwPoint_D_Rq/1(out) -> bus_creator/2  "ElPwPoint_D_Rq"
  HeadLghtHiPrmsn_D_Stat/1(out) -> bus_creator/3  "HeadLghtHiPrmsn_D_Stat"
  IgnPsswrdDsply_B_Rq/1(out) -> bus_creator/4  "IgnPsswrdDsply_B_Rq"
  KeyAdmnTot_No_Cnt/1(out) -> bus_creator/5  "KeyAdmnTot_No_Cnt"
  KeyMykeyTot_No_Cnt/1(out) -> bus_creator/6  "KeyMykeyTot_No_Cnt"
  Keycode_Status/1(out) -> bus_creator/7  "Keycode_Status"
  PEBackupSlot_Stats/1(out) -> bus_creator/8  "PEBackupSlot_Stats"
  PoliceIdlMde_D_Stat/1(out) -> bus_creator/9  "PoliceIdlMde_D_Stat"
  PrmtrAlrmEvnt_D_Stat/1(out) -> bus_creator/10  "PrmtrAlrmEvnt_D_Stat"
  PrsnlDevcChrgEnbl_B_Rq/1(out) -> bus_creator/11  "PrsnlDevcChrgEnbl_B_Rq"
  SecurityMsgTxt_D_Rq/1(out) -> bus_creator/12  "SecurityMsgTxt_D_Rq"
  SteWhlLckMsgTxt_D_Rq/1(out) -> bus_creator/13  "SteWhlLckMsgTxt_D_Rq"
  TracKeyMde_D_Stat/1(out) -> bus_creator/14  "TracKeyMde_D_Stat"
  immoMsgTxt_D_Rq/1(out) -> bus_creator/15  "immoMsgTxt_D_Rq"
  bus_selector/1 -> DrLatchMsgTxt_D_Rq/1(in)  "<DrLatchMsgTxt_D_Rq>"
  bus_selector/2 -> ElPwPoint_D_Rq/1(in)  "<ElPwPoint_D_Rq>"
  bus_selector/3 -> HeadLghtHiPrmsn_D_Stat/1(in)  "<HeadLghtHiPrmsn_D_Stat>"
  bus_selector/4 -> IgnPsswrdDsply_B_Rq/1(in)  "<IgnPsswrdDsply_B_Rq>"
  bus_selector/5 -> KeyAdmnTot_No_Cnt/1(in)  "<KeyAdmnTot_No_Cnt>"
  bus_selector/6 -> KeyMykeyTot_No_Cnt/1(in)  "<KeyMykeyTot_No_Cnt>"
  bus_selector/7 -> Keycode_Status/1(in)  "<Keycode_Status>"
  bus_selector/8 -> PEBackupSlot_Stats/1(in)  "<PEBackupSlot_Stats>"
  bus_selector/9 -> PoliceIdlMde_D_Stat/1(in)  "<PoliceIdlMde_D_Stat>"
  bus_selector/10 -> PrmtrAlrmEvnt_D_Stat/1(in)  "<PrmtrAlrmEvnt_D_Stat>"
  bus_selector/11 -> PrsnlDevcChrgEnbl_B_Rq/1(in)  "<PrsnlDevcChrgEnbl_B_Rq>"
  bus_selector/12 -> SecurityMsgTxt_D_Rq/1(in)  "<SecurityMsgTxt_D_Rq>"
  bus_selector/13 -> SteWhlLckMsgTxt_D_Rq/1(in)  "<SteWhlLckMsgTxt_D_Rq>"
  bus_selector/14 -> TracKeyMde_D_Stat/1(in)  "<TracKeyMde_D_Stat>"
  bus_selector/15 -> immoMsgTxt_D_Rq/1(in)  "<immoMsgTxt_D_Rq>"
  in/1 -> bus_selector/1

== system test_mdl_NI/CAN_Signal/GWM/Other_GWMTx/Body_Info_8_FD1 ==
  in : Inport
  ChrgCordLck_B_Stat : Subsystem
  ChrgCordResp1_No_Actl : Subsystem
  ChrgCordResp2_No_Actl : Subsystem
  WakeAlarm0_D_Stat : Subsystem
  WakeAlarm1_D_Stat : Subsystem
  WakeAlarm2_D_Stat : Subsystem
  WakeAlarm3_D_Stat : Subsystem
  bus_creator : BusCreator  Inputs=7
  bus_selector : BusSelector  OutputSignals=ChrgCordLck_B_Stat,ChrgCordResp1_No_Actl,ChrgCordResp2_No_Actl,WakeAlarm0_D_Stat,WakeAlarm1_D_Stat,WakeAlarm2_D_Stat,WakeAlarm3_D_Stat
  out_port : Outport
  wires:
  bus_creator/1 -> out_port/1  "Body_Info_8_FD1"
  ChrgCordLck_B_Stat/1(out) -> bus_creator/1  "ChrgCordLck_B_Stat"
  ChrgCordResp1_No_Actl/1(out) -> bus_creator/2  "ChrgCordResp1_No_Actl"
  ChrgCordResp2_No_Actl/1(out) -> bus_creator/3  "ChrgCordResp2_No_Actl"
  WakeAlarm0_D_Stat/1(out) -> bus_creator/4  "WakeAlarm0_D_Stat"
  WakeAlarm1_D_Stat/1(out) -> bus_creator/5  "WakeAlarm1_D_Stat"
  WakeAlarm2_D_Stat/1(out) -> bus_creator/6  "WakeAlarm2_D_Stat"
  WakeAlarm3_D_Stat/1(out) -> bus_creator/7  "WakeAlarm3_D_Stat"
  bus_selector/1 -> ChrgCordLck_B_Stat/1(in)  "<ChrgCordLck_B_Stat>"
  bus_selector/2 -> ChrgCordResp1_No_Actl/1(in)  "<ChrgCordResp1_No_Actl>"
  bus_selector/3 -> ChrgCordResp2_No_Actl/1(in)  "<ChrgCordResp2_No_Actl>"
  bus_selector/4 -> WakeAlarm0_D_Stat/1(in)  "<WakeAlarm0_D_Stat>"
  bus_selector/5 -> WakeAlarm1_D_Stat/1(in)  "<WakeAlarm1_D_Stat>"
  bus_selector/6 -> WakeAlarm2_D_Stat/1(in)  "<WakeAlarm2_D_Stat>"
  bus_selector/7 -> WakeAlarm3_D_Stat/1(in)  "<WakeAlarm3_D_Stat>"
  in/1 -> bus_selector/1

== system test_mdl_NI/CAN_Signal/GWM/Other_GWMTx/Body_Info_9_FD1 ==
  in : Inport
  AdvStrt_D_Stat : Subsystem
  CrnkInhbt_B_Stat : Subsystem
  CrnkInhbt_No_Cnt : Subsystem
  CrnkInhbt_No_Cs : Subsystem
  DrvInCtl_B_Stat : Subsystem
  EngStrtActv_B_Stat : Subsystem
  EngStrt_B_Rq : Subsystem
  IgnPreOffActv_B_Stat : Subsystem
  StrtrMtrCtlDStat_No_Cs : Subsystem
  VehOnSrc_D_Stat : Subsystem
  bus_creator : BusCreator  Inputs=10
  bus_selector : BusSelector  OutputSignals=AdvStrt_D_Stat,CrnkInhbt_B_Stat,CrnkInhbt_No_Cnt,CrnkInhbt_No_Cs,DrvInCtl_B_Stat,EngStrtActv_B_Stat,EngStrt_B_Rq,IgnPreOffActv_B_Stat,StrtrMtrCtlDStat_No_Cs,VehOnSrc_D_Stat
  out_port : Outport
  wires:
  bus_creator/1 -> out_port/1  "Body_Info_9_FD1"
  AdvStrt_D_Stat/1(out) -> bus_creator/1  "AdvStrt_D_Stat"
  CrnkInhbt_B_Stat/1(out) -> bus_creator/2  "CrnkInhbt_B_Stat"
  CrnkInhbt_No_Cnt/1(out) -> bus_creator/3  "CrnkInhbt_No_Cnt"
  CrnkInhbt_No_Cs/1(out) -> bus_creator/4  "CrnkInhbt_No_Cs"
  DrvInCtl_B_Stat/1(out) -> bus_creator/5  "DrvInCtl_B_Stat"
  EngStrtActv_B_Stat/1(out) -> bus_creator/6  "EngStrtActv_B_Stat"
  EngStrt_B_Rq/1(out) -> bus_creator/7  "EngStrt_B_Rq"
  IgnPreOffActv_B_Stat/1(out) -> bus_creator/8  "IgnPreOffActv_B_Stat"
  StrtrMtrCtlDStat_No_Cs/1(out) -> bus_creator/9  "StrtrMtrCtlDStat_No_Cs"
  VehOnSrc_D_Stat/1(out) -> bus_creator/10  "VehOnSrc_D_Stat"
  bus_selector/1 -> AdvStrt_D_Stat/1(in)  "<AdvStrt_D_Stat>"
  bus_selector/2 -> CrnkInhbt_B_Stat/1(in)  "<CrnkInhbt_B_Stat>"
  bus_selector/3 -> CrnkInhbt_No_Cnt/1(in)  "<CrnkInhbt_No_Cnt>"
  bus_selector/4 -> CrnkInhbt_No_Cs/1(in)  "<CrnkInhbt_No_Cs>"
  bus_selector/5 -> DrvInCtl_B_Stat/1(in)  "<DrvInCtl_B_Stat>"
  bus_selector/6 -> EngStrtActv_B_Stat/1(in)  "<EngStrtActv_B_Stat>"
  bus_selector/7 -> EngStrt_B_Rq/1(in)  "<EngStrt_B_Rq>"
  bus_selector/8 -> IgnPreOffActv_B_Stat/1(in)  "<IgnPreOffActv_B_Stat>"
  bus_selector/9 -> StrtrMtrCtlDStat_No_Cs/1(in)  "<StrtrMtrCtlDStat_No_Cs>"
  bus_selector/10 -> VehOnSrc_D_Stat/1(in)  "<VehOnSrc_D_Stat>"
  in/1 -> bus_selector/1

== system test_mdl_NI/CAN_Signal/GWM/Other_GWMTx/Climate_Cntrl_Data_2_FD1 ==
  in : Inport
  ApaSwtch_D_RqDrv : Subsystem
  ApaSwtch_No_Cnt : Subsystem
  CabnAmb_Te_Actl : Subsystem
  CamraDefog_B_Actl : Subsystem
  ClimtThrmlLoad_No_Actl : Subsystem
  EcoMde_D_RqDrv : Subsystem
  HvacAir_Flw_Est : Subsystem
  HvacBlwrFront_D_Stat : Subsystem
  HvacBlwrRear_D_Stat : Subsystem
  HvacRec_Pc_Est : Subsystem
  HvacRemoteStrt_N_Rq : Subsystem
  TwHlGrdAsst_B_RqTrn : Subsystem
  bus_creator : BusCreator  Inputs=12
  bus_selector : BusSelector  OutputSignals=ApaSwtch_D_RqDrv,ApaSwtch_No_Cnt,CabnAmb_Te_Actl,CamraDefog_B_Actl,ClimtThrmlLoad_No_Actl,EcoMde_D_RqDrv,HvacAir_Flw_Est,HvacBlwrFront_D_Stat,HvacBlwrRear_D_Stat,HvacRec_Pc_Est,HvacRemoteStrt_N_Rq,TwHlGrdAsst_B_RqTrn
  out_port : Outport
  wires:
  bus_creator/1 -> out_port/1  "Climate_Cntrl_Data_2_FD1"
  ApaSwtch_D_RqDrv/1(out) -> bus_creator/1  "ApaSwtch_D_RqDrv"
  ApaSwtch_No_Cnt/1(out) -> bus_creator/2  "ApaSwtch_No_Cnt"
  CabnAmb_Te_Actl/1(out) -> bus_creator/3  "CabnAmb_Te_Actl"
  CamraDefog_B_Actl/1(out) -> bus_creator/4  "CamraDefog_B_Actl"
  ClimtThrmlLoad_No_Actl/1(out) -> bus_creator/5  "ClimtThrmlLoad_No_Actl"
  EcoMde_D_RqDrv/1(out) -> bus_creator/6  "EcoMde_D_RqDrv"
  HvacAir_Flw_Est/1(out) -> bus_creator/7  "HvacAir_Flw_Est"
  HvacBlwrFront_D_Stat/1(out) -> bus_creator/8  "HvacBlwrFront_D_Stat"
  HvacBlwrRear_D_Stat/1(out) -> bus_creator/9  "HvacBlwrRear_D_Stat"
  HvacRec_Pc_Est/1(out) -> bus_creator/10  "HvacRec_Pc_Est"
  HvacRemoteStrt_N_Rq/1(out) -> bus_creator/11  "HvacRemoteStrt_N_Rq"
  TwHlGrdAsst_B_RqTrn/1(out) -> bus_creator/12  "TwHlGrdAsst_B_RqTrn"
  bus_selector/1 -> ApaSwtch_D_RqDrv/1(in)  "<ApaSwtch_D_RqDrv>"
  bus_selector/2 -> ApaSwtch_No_Cnt/1(in)  "<ApaSwtch_No_Cnt>"
  bus_selector/3 -> CabnAmb_Te_Actl/1(in)  "<CabnAmb_Te_Actl>"
  bus_selector/4 -> CamraDefog_B_Actl/1(in)  "<CamraDefog_B_Actl>"
  bus_selector/5 -> ClimtThrmlLoad_No_Actl/1(in)  "<ClimtThrmlLoad_No_Actl>"
  bus_selector/6 -> EcoMde_D_RqDrv/1(in)  "<EcoMde_D_RqDrv>"
  bus_selector/7 -> HvacAir_Flw_Est/1(in)  "<HvacAir_Flw_Est>"
  bus_selector/8 -> HvacBlwrFront_D_Stat/1(in)  "<HvacBlwrFront_D_Stat>"
  bus_selector/9 -> HvacBlwrRear_D_Stat/1(in)  "<HvacBlwrRear_D_Stat>"
  bus_selector/10 -> HvacRec_Pc_Est/1(in)  "<HvacRec_Pc_Est>"
  bus_selector/11 -> HvacRemoteStrt_N_Rq/1(in)  "<HvacRemoteStrt_N_Rq>"
  bus_selector/12 -> TwHlGrdAsst_B_RqTrn/1(in)  "<TwHlGrdAsst_B_RqTrn>"
  in/1 -> bus_selector/1

== system test_mdl_NI/CAN_Signal/GWM/Other_GWMTx/Climate_Control_Data_FD1 ==
  in : Inport
  AutoHoldSwtch_D_Stat : Subsystem
  CamraFrntBttn_D_Stat : Subsystem
  CamraRearBttn_D_Stat : Subsystem
  DrvSlipCtlMde_B_Rq : Subsystem
  EcoInhbt_B_RqHvac : Subsystem
  GlvBoxRleas_No_Actl : Subsystem
  LpdbAuxBlwr_B_Rq : Subsystem
  LpdbDfrstFlOn_B_Rq : Subsystem
  LpdbDfrstFrOn_B_Rq : Subsystem
  LpdbDfrstRearOn_B_Rq : Subsystem
  LpdbHeatWiprPrk_B_Rq : Subsystem
  LpdbPtc1_B_Rq : Subsystem
  LpdbPtc2_B_Rq : Subsystem
  LpdbPtc3_B_Rq : Subsystem
  MirrorHeatOn_B_Rq : Subsystem
  Outside_Air_Temp_Stat : Subsystem
  PrkAidSwtch_D_RqDrv : Subsystem
  PrkAidSwtch_No_Cnt : Subsystem
  Remote_Start_QuietMode : Subsystem
  SteWhlHeat_D_Rq : Subsystem
  TrailCtlSwtch_B_Stat : Subsystem
  bus_creator : BusCreator  Inputs=21
  bus_selector : BusSelector  OutputSignals=AutoHoldSwtch_D_Stat,CamraFrntBttn_D_Stat,CamraRearBttn_D_Stat,DrvSlipCtlMde_B_Rq,EcoInhbt_B_RqHvac,GlvBoxRleas_No_Actl,LpdbAuxBlwr_B_Rq,LpdbDfrstFlOn_B_Rq,LpdbDfrstFrOn_B_Rq,LpdbDfrstRearOn_B_Rq,LpdbHeatWiprPrk_B_Rq,LpdbPtc1_B_Rq,LpdbPtc2_B_Rq,LpdbPtc3_B_Rq,MirrorHeatOn_B_Rq,Outside_Air_Temp_Stat,PrkAidSwtch_D_RqDrv,PrkAidSwtch_No_Cnt,Remote_Start_QuietMode,SteWhlHeat_D_Rq,TrailCtlSwtch_B_Stat
  out_port : Outport
  wires:
  bus_creator/1 -> out_port/1  "Climate_Control_Data_FD1"
  AutoHoldSwtch_D_Stat/1(out) -> bus_creator/1  "AutoHoldSwtch_D_Stat"
  CamraFrntBttn_D_Stat/1(out) -> bus_creator/2  "CamraFrntBttn_D_Stat"
  CamraRearBttn_D_Stat/1(out) -> bus_creator/3  "CamraRearBttn_D_Stat"
  DrvSlipCtlMde_B_Rq/1(out) -> bus_creator/4  "DrvSlipCtlMde_B_Rq"
  EcoInhbt_B_RqHvac/1(out) -> bus_creator/5  "EcoInhbt_B_RqHvac"
  GlvBoxRleas_No_Actl/1(out) -> bus_creator/6  "GlvBoxRleas_No_Actl"
  LpdbAuxBlwr_B_Rq/1(out) -> bus_creator/7  "LpdbAuxBlwr_B_Rq"
  LpdbDfrstFlOn_B_Rq/1(out) -> bus_creator/8  "LpdbDfrstFlOn_B_Rq"
  LpdbDfrstFrOn_B_Rq/1(out) -> bus_creator/9  "LpdbDfrstFrOn_B_Rq"
  LpdbDfrstRearOn_B_Rq/1(out) -> bus_creator/10  "LpdbDfrstRearOn_B_Rq"
  LpdbHeatWiprPrk_B_Rq/1(out) -> bus_creator/11  "LpdbHeatWiprPrk_B_Rq"
  LpdbPtc1_B_Rq/1(out) -> bus_creator/12  "LpdbPtc1_B_Rq"
  LpdbPtc2_B_Rq/1(out) -> bus_creator/13  "LpdbPtc2_B_Rq"
  LpdbPtc3_B_Rq/1(out) -> bus_creator/14  "LpdbPtc3_B_Rq"
  MirrorHeatOn_B_Rq/1(out) -> bus_creator/15  "MirrorHeatOn_B_Rq"
  Outside_Air_Temp_Stat/1(out) -> bus_creator/16  "Outside_Air_Temp_Stat"
  PrkAidSwtch_D_RqDrv/1(out) -> bus_creator/17  "PrkAidSwtch_D_RqDrv"
  PrkAidSwtch_No_Cnt/1(out) -> bus_creator/18  "PrkAidSwtch_No_Cnt"
  Remote_Start_QuietMode/1(out) -> bus_creator/19  "Remote_Start_QuietMode"
  SteWhlHeat_D_Rq/1(out) -> bus_creator/20  "SteWhlHeat_D_Rq"
  TrailCtlSwtch_B_Stat/1(out) -> bus_creator/21  "TrailCtlSwtch_B_Stat"
  bus_selector/1 -> AutoHoldSwtch_D_Stat/1(in)  "<AutoHoldSwtch_D_Stat>"
  bus_selector/2 -> CamraFrntBttn_D_Stat/1(in)  "<CamraFrntBttn_D_Stat>"
  bus_selector/3 -> CamraRearBttn_D_Stat/1(in)  "<CamraRearBttn_D_Stat>"
  bus_selector/4 -> DrvSlipCtlMde_B_Rq/1(in)  "<DrvSlipCtlMde_B_Rq>"
  bus_selector/5 -> EcoInhbt_B_RqHvac/1(in)  "<EcoInhbt_B_RqHvac>"
  bus_selector/6 -> GlvBoxRleas_No_Actl/1(in)  "<GlvBoxRleas_No_Actl>"
  bus_selector/7 -> LpdbAuxBlwr_B_Rq/1(in)  "<LpdbAuxBlwr_B_Rq>"
  bus_selector/8 -> LpdbDfrstFlOn_B_Rq/1(in)  "<LpdbDfrstFlOn_B_Rq>"
  bus_selector/9 -> LpdbDfrstFrOn_B_Rq/1(in)  "<LpdbDfrstFrOn_B_Rq>"
  bus_selector/10 -> LpdbDfrstRearOn_B_Rq/1(in)  "<LpdbDfrstRearOn_B_Rq>"
  bus_selector/11 -> LpdbHeatWiprPrk_B_Rq/1(in)  "<LpdbHeatWiprPrk_B_Rq>"
  bus_selector/12 -> LpdbPtc1_B_Rq/1(in)  "<LpdbPtc1_B_Rq>"
  bus_selector/13 -> LpdbPtc2_B_Rq/1(in)  "<LpdbPtc2_B_Rq>"
  bus_selector/14 -> LpdbPtc3_B_Rq/1(in)  "<LpdbPtc3_B_Rq>"
  bus_selector/15 -> MirrorHeatOn_B_Rq/1(in)  "<MirrorHeatOn_B_Rq>"
  bus_selector/16 -> Outside_Air_Temp_Stat/1(in)  "<Outside_Air_Temp_Stat>"
  bus_selector/17 -> PrkAidSwtch_D_RqDrv/1(in)  "<PrkAidSwtch_D_RqDrv>"
  bus_selector/18 -> PrkAidSwtch_No_Cnt/1(in)  "<PrkAidSwtch_No_Cnt>"
  bus_selector/19 -> Remote_Start_QuietMode/1(in)  "<Remote_Start_QuietMode>"
  bus_selector/20 -> SteWhlHeat_D_Rq/1(in)  "<SteWhlHeat_D_Rq>"
  bus_selector/21 -> TrailCtlSwtch_B_Stat/1(in)  "<TrailCtlSwtch_B_Stat>"
  in/1 -> bus_selector/1
